simulink model "WT_FAST_09_07_2023_Afzalian"  (R2015b)
settings: Solver=FixedStepAuto  StartTime=0.0  StopTime=TMax  FixedStep=DT  MaxStep=DT  RelTol=1e-3
undefined symbols (not defined in the file): NDOF, NumOuts, q_init, qdot_init, TMax, wn, wn_A, wn_H, wn_P, zeta, zeta_A, zeta_H, zeta_P
settings Model: Creator=bjonkman  LastModifiedBy=SBU
settings SolverCC: AlgebraicLoopSolver=LineSearch
settings DataIOCC: LimitDataPoints=off  SaveFormat=Array  SignalLoggingSaveFormat=ModelDataLogs  SaveOutput=off  SaveTime=off  SignalLoggingName=sigsOut
settings OptimizationCC: ExpressionDepthLimit=2147483647
settings DebuggingCC: SaveWithParameterizedLinksMsg=none  UnderspecifiedInitializationDetection=Classic  MergeDetectMultiDrivingBlocksExec=none  SignalResolutionControl=TryResolveAllWithWarning  MultiTaskDSMMsg=warning  MultiTaskCondExecSysMsg=none  FcnCallInpInsideContextMsg=UseLocalSettings  StateNameClashWarn=warning
settings HardwareCC: ProdBitPerPointer=32  ProdLargestAtomicFloat=None  ProdIntDivRoundTo=Undefined  ProdEndianess=Unspecified  ProdWordSize=32  ProdHWDeviceType=32-bit Generic  TargetUnknown=on
settings GRTTargetCC: ModelReferenceCompliant=off  ParMdlRefBuildCompliant=off  CompOptLevelCompliant=off  ConcurrentExecutionCompliant=off  GeneratePreprocessorConditionals=Disable all  CombineOutputUpdateFcns=off  MatFileLogging=off  MATLABClassNameForMDSCustomization=Simulink.SoftwareTarget.TargetSpecificTriggerConfigurationBase  GRTInterface=on
settings ConfigComp: CovModelRefEnable=Off  CovSFcnEnable=off

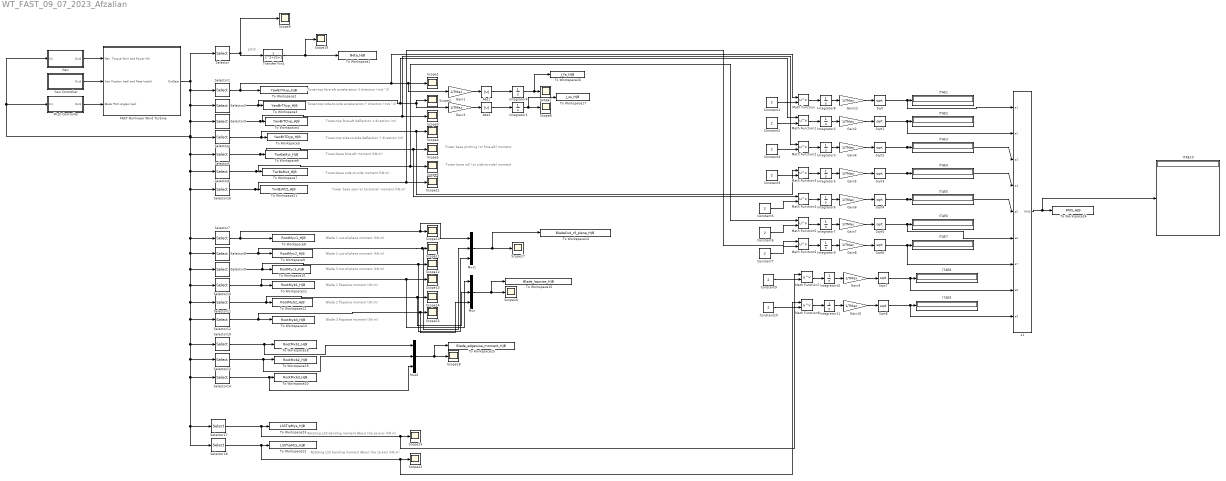
== system WT_FAST_09_07_2023_Afzalian ==
  note: Tower base yaw (or torsional) moment (kN.m)
  note: Tower base pitching (or fore-aft) moment
  note: Tower base roll (or side-to-side) moment
  note: Tower-base side-to-side moment (kN.m)
  note: Tower-base fore-aft moment (kN.m)
  note: Tower-top side-to-side deflection Y direction (m)
  note: Tower-top fore-aft deflection X direction (m)
  note: pitch
  note: Tower-top fore-aft acceleration X direction (m/s^2)
  note: Tower-top side-to-side acceleration Y direction (m/s^2)
  note: Blade 3 flapwise moment (kN.m)
  note: Blade 2 flapwise moment (kN.m)
  note: Blade 1 flapwise moment (kN.m)
  note: Blade 3 out-of-plane moment (kN.m)
  note: Blade 1 out-of-plane moment (kN.m)
  note: Blade 2 out-of-plane moment (kN.m)
  note: Rotating LSS bending moment About the ya-axis (kN.m)
  note: Rotating LSS bending moment About the za-axis (kN.m)
  Abs1 : Abs
  Abs2 : Abs
  Constant{1..7,9..10} (9 alike) : Constant  Value=2
  FAST Nonlinear Wind Turbine : Subsystem  mask(FAST Nonlinear Wind Turbine){}
      mask help: This block contains the FAST S-Function and blocks that integrate the DOF accelerations to get velocities and displacements.
      mask init:
      | clear FAST_SFunc
  Gain{1..10,12} (11 alike) : Gain  Gain=1/TMax
  Gen : Subsystem
  ITAE{1..10} (10 alike) : Display
  Integrator1 : Integrator  UpperSaturationLimit=5  LowerSaturationLimit=-5
  Integrator{2..3,5..11} (9 alike) : Integrator  UpperSaturationLimit=0.2  LowerSaturationLimit=-0.2
  Integrator4 : Integrator  UpperSaturationLimit=5  LowerSaturationLimit=-5
  Math Function{,1..8} (9 alike) : Math  Operator=pow  SaturateOnIntegerOverflow=on
  Mux : Mux  Inputs=3
  Mux1 : Mux  Inputs=3
  Mux2 : Mux  Inputs=3
  Pitch Controller : Subsystem
  Scope{1..19,21..23} (22 alike) : Scope
  Selector : Selector  InputPortWidth=48  IndexOptions=Index vector (dialog)  Indices=[9]  OutputSizes=1
  Selector1 : Selector  InputPortWidth=48  IndexOptions=Index vector (dialog)  Indices=[31]  OutputSizes=1
  Selector10 : Selector  InputPortWidth=48  IndexOptions=Index vector (dialog)  Indices=[41]  OutputSizes=1
  Selector11 : Selector  InputPortWidth=48  IndexOptions=Index vector (dialog)  Indices=[42]  OutputSizes=1
  Selector12 : Selector  InputPortWidth=48  IndexOptions=Index vector (dialog)  Indices=[43]  OutputSizes=1
  Selector13 : Selector  InputPortWidth=48  IndexOptions=Index vector (dialog)  Indices=[45]  OutputSizes=1
  Selector14 : Selector  InputPortWidth=48  IndexOptions=Index vector (dialog)  Indices=[46]  OutputSizes=1
  Selector16 : Selector  InputPortWidth=48  IndexOptions=Index vector (dialog)  Indices=[37]  OutputSizes=1
  Selector17 : Selector  InputPortWidth=48  IndexOptions=Index vector (dialog)  Indices=[44]  OutputSizes=1
  Selector18 : Selector  InputPortWidth=48  IndexOptions=Index vector (dialog)  Indices=[45]  OutputSizes=1
  Selector19 : Selector  InputPortWidth=48  IndexOptions=Index vector (dialog)  Indices=[44]  OutputSizes=1
  Selector2 : Selector  InputPortWidth=48  IndexOptions=Index vector (dialog)  Indices=[32]  OutputSizes=1
  Selector3 : Selector  InputPortWidth=48  IndexOptions=Index vector (dialog)  Indices=[33]  OutputSizes=1
  Selector4 : Selector  InputPortWidth=48  IndexOptions=Index vector (dialog)  Indices=[34]  OutputSizes=1
  Selector5 : Selector  InputPortWidth=48  IndexOptions=Index vector (dialog)  Indices=[35]  OutputSizes=1
  Selector6 : Selector  InputPortWidth=48  IndexOptions=Index vector (dialog)  Indices=[36]  OutputSizes=1
  Selector7 : Selector  InputPortWidth=48  IndexOptions=Index vector (dialog)  Indices=[38]  OutputSizes=1
  Selector8 : Selector  InputPortWidth=48  IndexOptions=Index vector (dialog)  Indices=[39]  OutputSizes=1
  Selector9 : Selector  InputPortWidth=48  IndexOptions=Index vector (dialog)  Indices=[40]  OutputSizes=1
  Sqrt{,1..8} (9 alike) : Sqrt  SaturateOnIntegerOverflow=on
  To Workspace1 : ToWorkspace  VariableName=Beta_HJB  SaveFormat=Structure With Time  SampleTime=-1
  To Workspace10 : ToWorkspace  VariableName=RootMyc3_HJB  SaveFormat=Structure With Time  SampleTime=-1
  To Workspace11 : ToWorkspace  VariableName=RootMyb1_HJB  SaveFormat=Structure With Time  SampleTime=-1
  To Workspace12 : ToWorkspace  VariableName=RootMyb2_HJB  SaveFormat=Structure With Time  SampleTime=-1
  To Workspace13 : ToWorkspace  VariableName=RootMyb3_HJB  SaveFormat=Structure With Time  SampleTime=-1
  To Workspace14 : ToWorkspace  VariableName=BladeOut_of_plane_HJB  SaveFormat=Structure With Time  SampleTime=-1
  To Workspace15 : ToWorkspace  VariableName=Blade_lapwise_HJB  SaveFormat=Structure With Time  SampleTime=-1
  To Workspace16 : ToWorkspace  VariableName=J_fa_HJB  SaveFormat=Structure With Time  SampleTime=-1
  To Workspace17 : ToWorkspace  VariableName=J_ss_HJB  SaveFormat=Structure With Time  SampleTime=-1
  To Workspace18 : ToWorkspace  VariableName=RootMxb1_HJB  SaveFormat=Structure With Time  SampleTime=-1
  To Workspace19 : ToWorkspace  VariableName=RootMxb2_HJB  SaveFormat=Structure With Time  SampleTime=-1
  To Workspace2 : ToWorkspace  VariableName=YawBrTAxp_HJB  SaveFormat=Structure With Time  SampleTime=-1
  To Workspace20 : ToWorkspace  VariableName=RootMxb3_HJB  SaveFormat=Structure With Time  SampleTime=-1
  To Workspace21 : ToWorkspace  VariableName=TwrBsMzt_HJB  SaveFormat=Structure With Time  SampleTime=-1
  To Workspace22 : ToWorkspace  VariableName=LSSTipMzs_HJB  SaveFormat=Structure With Time  SampleTime=-1
  To Workspace23 : ToWorkspace  VariableName=LSSTipMys_HJB  SaveFormat=Structure With Time  SampleTime=-1
  To Workspace24 : ToWorkspace  VariableName=RMS_HJB  SaveFormat=Structure With Time  SampleTime=-1
  To Workspace25 : ToWorkspace  VariableName=Blade_edgewise_moment_HJB  SaveFormat=Structure With Time  SampleTime=-1
  To Workspace3 : ToWorkspace  VariableName=YawBrTAyp_HJB  SaveFormat=Structure With Time  SampleTime=-1
  To Workspace4 : ToWorkspace  VariableName=YawBrTDxp_HJB  SaveFormat=Structure With Time  SampleTime=-1
  To Workspace5 : ToWorkspace  VariableName=YawBrTDyp_HJB  SaveFormat=Structure With Time  SampleTime=-1
  To Workspace6 : ToWorkspace  VariableName=TwrBsMyt_HJB  SaveFormat=Structure With Time  SampleTime=-1
  To Workspace7 : ToWorkspace  VariableName=TwrBsMxt_HJB  SaveFormat=Structure With Time  SampleTime=-1
  To Workspace8 : ToWorkspace  VariableName=RootMyc1_HJB  SaveFormat=Structure With Time  SampleTime=-1
  To Workspace9 : ToWorkspace  VariableName=RootMyc2_HJB  SaveFormat=Structure With Time  SampleTime=-1
  Transfer Fcn1 : TransferFcn
  Yaw Controller : Subsystem
  s1 : MATLAB Function  TreatAsAtomicUnit=on
  wires:
  Yaw Controller/1(Out1) -> FAST Nonlinear Wind Turbine/2(Yaw Position (rad) and Rate (rad/s))
  Pitch Controller/1(Out1) -> FAST Nonlinear Wind Turbine/3(Blade Pitch Angles (rad))
  Gen/1(Out1) -> FAST Nonlinear Wind Turbine/1(Gen. Torque (Nm) and Power (W))
  Selector9/1 -> To Workspace10/1, Mux1/3, Scope12/1
  Selector10/1 -> To Workspace11/1, Mux/1, Scope13/1
  Selector12/1 -> To Workspace13/1, Mux/3, Scope15/1
  Selector8/1 -> To Workspace9/1, Mux1/2, Scope11/1
  Selector7/1 -> To Workspace8/1, Mux1/1, Scope10/1
  Selector11/1 -> To Workspace12/1, Mux/2, Scope14/1
  Mux/1 -> To Workspace15/1, Scope16/1
  Mux1/1 -> To Workspace14/1, Scope17/1
  Abs1/1 -> Integrator4/1
  Abs2/1 -> Integrator1/1
  Integrator1/1 -> To Workspace17/1, Scope8/1
  Integrator4/1 -> To Workspace16/1, Scope7/1
  Gain1/1 -> Abs1/1
  Gain3/1 -> Abs2/1
  Selector18/1 -> To Workspace22/1, Math Function8/1, Scope22/1
  Selector17/1 -> Math Function7/1, Scope23/1, To Workspace23/1
  Selector4/1 -> Math Function3/1, Scope4/1, To Workspace5/1
  Selector5/1 -> Math Function4/1, Scope5/1, To Workspace6/1
  Selector1/1 -> Math Function/1, Gain1/1, Scope1/1, To Workspace2/1
  Math Function/1 -> Integrator8/1
  Constant1/1 -> Math Function/2
  Integrator8/1 -> Gain12/1
  Gain12/1 -> Sqrt/1
  Selector2/1 -> Math Function1/1, Gain3/1, Scope2/1, To Workspace3/1
  Math Function1/1 -> Integrator2/1
  Constant2/1 -> Math Function1/2
  Integrator2/1 -> Gain2/1
  Gain2/1 -> Sqrt1/1
  Selector3/1 -> Math Function2/1, Scope3/1, To Workspace4/1
  Math Function2/1 -> Integrator3/1
  Constant4/1 -> Math Function2/2
  Integrator3/1 -> Gain4/1
  Gain4/1 -> Sqrt2/1
  Math Function3/1 -> Integrator5/1
  Constant3/1 -> Math Function3/2
  Integrator5/1 -> Gain5/1
  Gain5/1 -> Sqrt3/1
  Constant5/1 -> Math Function4/2
  Gain6/1 -> Sqrt4/1
  Selector6/1 -> Math Function5/1, Scope6/1, To Workspace7/1
  Constant6/1 -> Math Function5/2
  Gain7/1 -> Sqrt5/1
  Integrator7/1 -> Gain7/1
  Integrator6/1 -> Gain6/1
  Math Function4/1 -> Integrator6/1
  Math Function5/1 -> Integrator7/1
  Selector16/1 -> Math Function6/1, Scope21/1, To Workspace21/1
  Constant7/1 -> Math Function6/2
  Gain8/1 -> Sqrt6/1
  Integrator9/1 -> Gain8/1
  Math Function6/1 -> Integrator9/1
  Sqrt/1 -> s1/1(a1), ITAE1/1
  Sqrt1/1 -> s1/2(a2), ITAE2/1
  Sqrt2/1 -> s1/3(a3), ITAE3/1
  Sqrt3/1 -> s1/4(a4), ITAE4/1
  Sqrt4/1 -> s1/5(a5), ITAE5/1
  Sqrt6/1 -> s1/7(a7), ITAE7/1
  s1/1(RMS) -> ITAE10/1, To Workspace24/1
  Sqrt5/1 -> s1/6(a6), ITAE6/1
  Constant9/1 -> Math Function7/2
  Gain9/1 -> Sqrt7/1
  Integrator10/1 -> Gain9/1
  Math Function7/1 -> Integrator10/1
  Sqrt7/1 -> s1/8(a8), ITAE8/1
  Constant10/1 -> Math Function8/2
  Gain10/1 -> Sqrt8/1
  Integrator11/1 -> Gain10/1
  Math Function8/1 -> Integrator11/1
  Sqrt8/1 -> s1/9(a9), ITAE9/1
  FAST Nonlinear Wind Turbine/1(OutData) -> Selector16/1, Selector19/1, Selector13/1, Selector14/1, Selector18/1, Selector17/1, Selector12/1, Selector11/1, Selector10/1, Selector9/1, Selector8/1, Selector7/1, Selector6/1, Selector5/1, Selector4/1, Gen/1(In1), Pitch Controller/1(In1), Selector3/1, Selector2/1, Selector1/1, Selector/1
  Selector19/1 -> Mux2/1, To Workspace18/1
  Selector13/1 -> Mux2/2, To Workspace19/1
  Selector14/1 -> Mux2/3, To Workspace20/1
  Mux2/1 -> Scope18/1, To Workspace25/1
  Selector/1 -> Transfer Fcn1/1, Scope9/1
  Transfer Fcn1/1 -> Scope19/1, To Workspace1/1

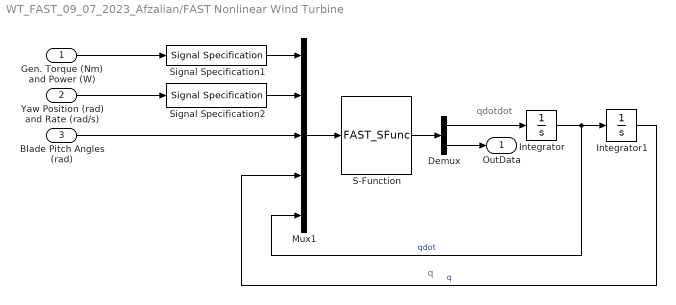
== system WT_FAST_09_07_2023_Afzalian/FAST Nonlinear Wind Turbine ==
  note: qdotdot
  note: q
  Gen. Torque (Nm) and Power (W) : Inport
  Yaw Position (rad) and Rate (rad/s) : Inport  Port=2
  Blade Pitch Angles (rad) : Inport  Port=3
  Demux : Demux  Outputs=[NDOF, NumOuts]
  Integrator : Integrator  InitialCondition=qdot_init
  Integrator1 : Integrator  InitialCondition=q_init
  Mux1 : Mux  Inputs=5
  S-Function : S-Function  FunctionName=FAST_SFunc  SFunctionDeploymentMode=off  EnableBusSupport=off
  Signal Specification1 : SignalSpecification  OutDataTypeStr=double  Dimensions=2
  Signal Specification2 : SignalSpecification  OutDataTypeStr=double  Dimensions=2
  OutData : Outport
  wires:
  Integrator/1 -> Integrator1/1, Mux1/5  "qdot"
  Gen. Torque (Nm) and Power (W)/1 -> Signal Specification1/1
  S-Function/1 -> Demux/1
  Demux/1 -> Integrator/1
  Demux/2 -> OutData/1
  Mux1/1 -> S-Function/1
  Blade Pitch Angles (rad)/1 -> Mux1/3
  Yaw Position (rad) and Rate (rad/s)/1 -> Signal Specification2/1
  Integrator1/1 -> Mux1/4  "q"
  Signal Specification1/1 -> Mux1/1
  Signal Specification2/1 -> Mux1/2

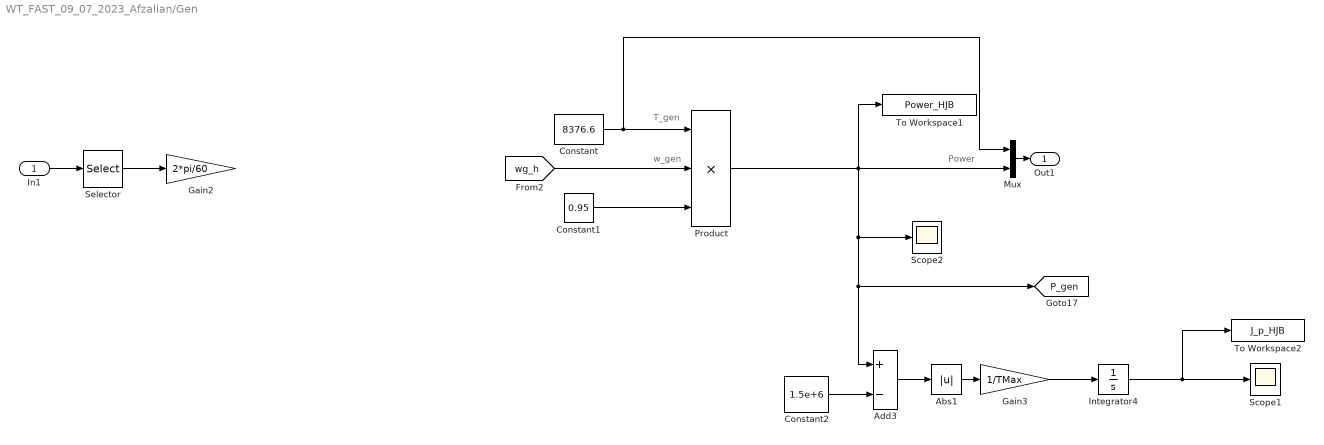
== system WT_FAST_09_07_2023_Afzalian/Gen ==
  note: T_gen
  note: w_gen
  note: Power
  In1 : Inport
  Abs1 : Abs
  Add3 : Sum  Inputs=+-
  Constant : Constant  Value=8376.6
  Constant1 : Constant  Value=0.95
  Constant2 : Constant  Value=1.5e+6
  Gain2 : Gain  Gain=2*pi/60
  Gain3 : Gain  Gain=1/TMax
  Integrator4 : Integrator  UpperSaturationLimit=5  LowerSaturationLimit=-5
  Mux : Mux  Inputs=2
  Product : Product  Inputs=3
  Scope1 : Scope
  Scope2 : Scope
  Selector : Selector  InputPortWidth=48  IndexOptions=Index vector (dialog)  Indices=[25]  OutputSizes=1
  To Workspace1 : ToWorkspace  VariableName=Power_HJB  SaveFormat=Structure With Time  SampleTime=-1
  To Workspace2 : ToWorkspace  VariableName=J_p_HJB  SaveFormat=Structure With Time  SampleTime=-1
  Out1 : Outport
  tag scope: P_gen=global
  wires:
  Constant1/1 -> Product/3
  Constant/1 -> Mux/1, Product/1
  In1/1 -> Selector/1
  Selector/1 -> Gain2/1
  Product/1 -> To Workspace1/1, Mux/2, Add3/1, [P_gen], Scope2/1
  Constant2/1 -> Add3/2
  Add3/1 -> Abs1/1
  Integrator4/1 -> Scope1/1, To Workspace2/1
  Gain3/1 -> Integrator4/1
  Abs1/1 -> Gain3/1
  Mux/1 -> Out1/1
  [wg_h] -> Product/2

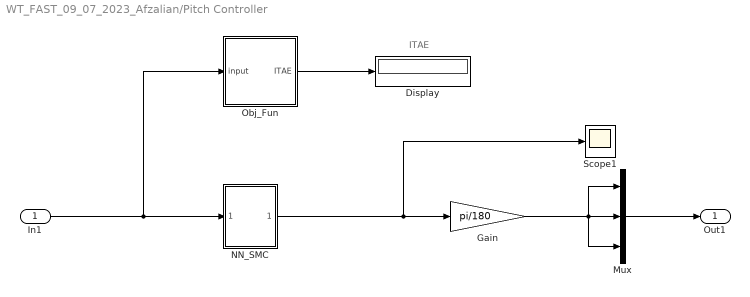
== system WT_FAST_09_07_2023_Afzalian/Pitch Controller ==
  note: ITAE
  In1 : Inport
  Display : Display
  Gain : Gain  Gain=pi/180
  Mux : Mux  Inputs=3
  NN_SMC : Subsystem
  Obj_Fun : Subsystem
  Scope1 : Scope
  Out1 : Outport
  wires:
  In1/1 -> NN_SMC/1(input), Obj_Fun/1("input ")
  Obj_Fun/1(ITAE) -> Display/1
  Mux/1 -> Out1/1
  Gain/1 -> Mux/3, Mux/1, Mux/2
  NN_SMC/1(Out1) -> Scope1/1, Gain/1

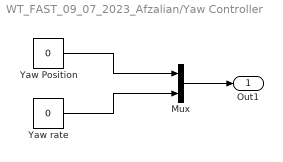
== system WT_FAST_09_07_2023_Afzalian/Yaw Controller ==
  Mux : Mux  Inputs=2
  Yaw Position : Constant  Value=0
  Yaw rate : Constant  Value=0
  Out1 : Outport
  wires:
  Mux/1 -> Out1/1
  Yaw Position/1 -> Mux/1
  Yaw rate/1 -> Mux/2

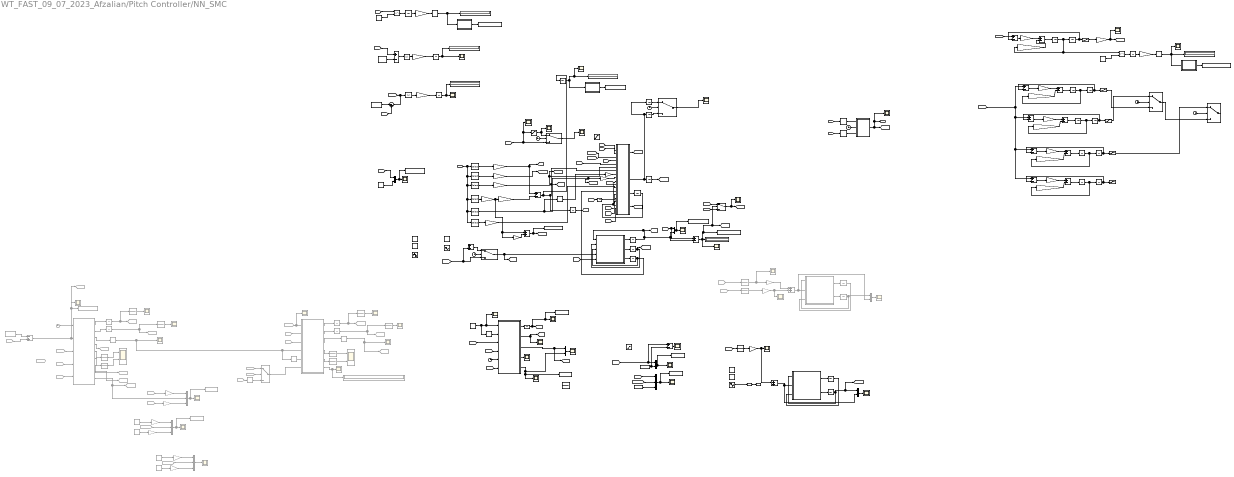
== system WT_FAST_09_07_2023_Afzalian/Pitch Controller/NN_SMC ==
  note: Step 1
  note: wind
  note: deltadot
  note: wgen
  note: xdot2
  note: xdot1
  note: w_rotor
  note: Step 2
  note: Stress
  note: J_P
  note: RMSE
  note: J_w
  input : Inport
  Abs1 : Abs
  Abs6 : Abs
  Add{,1,4,7,9..13,15..19} (14 alike) : Sum  Inputs=+-
  Add14 : Sum
  Add2 : Sum  Commented=on
  Add3 : Sum
  Add5 : Sum
  Add6 : Sum  Commented=on  Inputs=-+
  Clock{1..2,4..8} (7 alike) : Clock
  Clock3 : Clock  Commented=on
  Constant10 : Constant
  Constant11 : Constant  Value=rand
  Constant12 : Constant  Value=0.5
  Constant13 : Constant
  Constant14 : Constant  Value=1.5e6
  Constant15 : Constant
  Constant2 : Constant  Value=2
  Constant3 : Constant  Value=2
  Constant4 : Constant  Value=rand
  Constant5 : Constant  Commented=on  Value=1.5
  Constant6 : Constant  Commented=on  Value=0.5
  Constant7 : Constant  Commented=on  Value=0.5
  Constant8 : Constant  Commented=on  Value=1.5
  Constant9 : Constant  Value=1.5e+6
  D_hat : MATLAB Function  Commented=on  TreatAsAtomicUnit=on
  D_hat1 : MATLAB Function  TreatAsAtomicUnit=on
  Delay : Delay  DelayLength=1  InitialCondition=0
  Delay1 : Delay  DelayLength=1  InitialCondition=0
  Derivative{,1..2,4} (4 alike) : Derivative
  Derivative3 : Derivative  Commented=on
  Display : Display
  From14 : From  Commented=on  GotoTag=W_c  TagVisibility=global
  From15 : From  Commented=on  GotoTag=WWW  TagVisibility=global
  From17 : From  Commented=on  GotoTag=V  TagVisibility=global
  From31 : From  Commented=on  GotoTag=xdot1  TagVisibility=global
  From32 : From  Commented=on  GotoTag=W_a  TagVisibility=global
  From33 : From  Commented=on  GotoTag=W2_c  TagVisibility=global
  From35 : From  Commented=on  GotoTag=Res  TagVisibility=global
  From36 : From  Commented=on  GotoTag=wdotr_hat  TagVisibility=global
  From37 : From  Commented=on  GotoTag=wdotr_hat  TagVisibility=global
  From38 : From  Commented=on  GotoTag=rho_U  TagVisibility=global
  From39 : From  Commented=on  GotoTag=EE  TagVisibility=global
  From40 : From  Commented=on  GotoTag=W2_a  TagVisibility=global
  From41 : From  Commented=on  GotoTag=F_h  TagVisibility=global
  From42 : From  Commented=on  GotoTag=Lf  TagVisibility=global
  From44 : From  Commented=on  GotoTag=rho_L  TagVisibility=global
  From45 : From  Commented=on  GotoTag=EE  TagVisibility=global
  From6 : From  Commented=on  GotoTag=Lf  TagVisibility=global
  Gain : Gain  Gain=2*pi/60
  Gain1 : Gain  Gain=pi/180
  Gain{5,8,10,25} (4 alike) : Gain  Commented=on
  Gain{11,17,19..20} (4 alike) : Gain
  Gain{12,14..15,23} (4 alike) : Gain  Gain=1/TMax
  Gain13 : Gain  Gain=2*zeta*wn
  Gain16 : Gain  Gain=0.01
  Gain18 : Gain  Commented=on  Gain=0.3
  Gain2 : Gain  Gain=pi/180
  Gain21 : Gain  Commented=on  Gain=-1
  Gain22 : Gain  Commented=on  Gain=-1
  Gain24 : Gain  Commented=on  Gain=-1
  Gain26 : Gain  Gain=2*zeta_A*wn_A
  Gain27 : Gain  Gain=wn_P
  Gain28 : Gain  Gain=2*zeta_P*wn_P
  Gain29 : Gain  Gain=wn
  Gain3 : Gain  Gain=2*pi/60
  Gain30 : Gain  Gain=2*zeta*wn
  Gain31 : Gain  Gain=wn_H
  Gain32 : Gain  Gain=2*zeta_H*wn_H
  Gain4 : Gain  Gain=1/87.965
  Gain6 : Gain  Gain=1000
  Gain7 : Gain  Gain=wn
  Gain9 : Gain  Gain=wn_A
  Goto15 : Goto  Commented=on  GotoTag=W2_a  TagVisibility=global
  Goto16 : Goto  Commented=on  GotoTag=W_a  TagVisibility=global
  Goto2 : Goto  Commented=on  GotoTag=S  TagVisibility=global
  Goto23 : Goto  Commented=on  GotoTag=EE  TagVisibility=global
  Goto24 : Goto  Commented=on  GotoTag=YY  TagVisibility=global
  Goto25 : Goto  Commented=on  GotoTag=rho_U  TagVisibility=global
  Goto26 : Goto  Commented=on  GotoTag=W2_c  TagVisibility=global
  Goto27 : Goto  Commented=on  GotoTag=rho_L  TagVisibility=global
  Goto28 : Goto  Commented=on  GotoTag=W_c  TagVisibility=global
  Goto29 : Goto  Commented=on  GotoTag=e_1  TagVisibility=global
  ITAE{1,3..6} (5 alike) : Display
  ITAE2 : Display  Commented=on
  Integrator1 : Integrator  UpperSaturationLimit=5  LowerSaturationLimit=-5
  Integrator{8..10,14} (4 alike) : Integrator  Commented=on  InitialCondition=0.1  UpperSaturationLimit=10  LowerSaturationLimit=-10
  Integrator11 : Integrator  Commented=on  InitialCondition=0.1
  Integrator12 : Integrator  InitialCondition=0.1  LimitOutput=on  UpperSaturationLimit=100  LowerSaturationLimit=-100
  Integrator13 : Integrator  InitialCondition=0.1  UpperSaturationLimit=10  LowerSaturationLimit=-10
  Integrator{2,6,15,25,27,29} (6 alike) : Integrator  UpperSaturationLimit=90  LowerSaturationLimit=-1
  Integrator16 : Integrator  InitialCondition=2.1428
  Integrator17 : Integrator  Commented=on  InitialCondition=0.1
  Integrator18 : Integrator
  Integrator{19,26,28,30..31} (5 alike) : Integrator  LimitOutput=on  UpperSaturationLimit=8  LowerSaturationLimit=-8
  Integrator20 : Integrator  UpperSaturationLimit=0.2  LowerSaturationLimit=-0.2
  Integrator21 : Integrator  UpperSaturationLimit=0.2  LowerSaturationLimit=-0.2
  Integrator22 : Integrator  InitialCondition=180  LimitOutput=on  UpperSaturationLimit=200  LowerSaturationLimit=170
  Integrator23 : Integrator
  Integrator24 : Integrator  UpperSaturationLimit=5  LowerSaturationLimit=-5
  Integrator3 : Integrator  InitialCondition=2.1428  UpperSaturationLimit=2.5
  Integrator32 : Integrator  InitialCondition=0.1  UpperSaturationLimit=500  LowerSaturationLimit=-500
  Integrator33 : Integrator  UpperSaturationLimit=200
  Integrator4 : Integrator  UpperSaturationLimit=0.2  LowerSaturationLimit=-0.2
  Integrator5 : Integrator  UpperSaturationLimit=10  LowerSaturationLimit=-10
  Integrator7 : Integrator  InitialCondition=0.3
  Math Function1 : Math  Operator=pow  SaturateOnIntegerOverflow=on
  Math Function2 : Math  Operator=pow  SaturateOnIntegerOverflow=on
  Memory2 : Memory  Commented=on
  Memory3 : Memory  Commented=on
  Memory4 : Memory  Commented=on
  Mux{,1,4..5,9} (5 alike) : Mux  Inputs=2
  Mux2 : Mux  Commented=on  Inputs=2
  Mux3 : Mux  Inputs=3
  Mux6 : Mux  Commented=on  Inputs=3
  Mux7 : Mux  Commented=on  Inputs=3
  Mux8 : Mux  Commented=on  Inputs=3
  Observer1 : MATLAB Function  TreatAsAtomicUnit=on
  Observer2 : MATLAB Function  TreatAsAtomicUnit=on
  Observer3 : MATLAB Function  TreatAsAtomicUnit=on
  Observer4 : MATLAB Function  TreatAsAtomicUnit=on
  SMC : MATLAB Function  TreatAsAtomicUnit=on
  Saturation{1,4..7} (5 alike) : Saturate  UpperLimit=90  LowerLimit=-1
  Saturation2 : Saturate  UpperLimit=2.2  LowerLimit=-2.2
  Saturation3 : Saturate  UpperLimit=2.2  LowerLimit=-2.2
  Saturation9 : Saturate  UpperLimit=200  LowerLimit=-200
  Scope{1..4,6..7,9} (7 alike) : Scope
  Selector : Selector  InputPortWidth=48  IndexOptions=Index vector (dialog)  Indices=[24]  OutputSizes=1
  Selector1 : Selector  InputPortWidth=48  IndexOptions=Index vector (dialog)  Indices=[29]  OutputSizes=1
  Selector2 : Selector  InputPortWidth=48  IndexOptions=Index vector (dialog)  Indices=[30]  OutputSizes=1
  Selector3 : Selector  InputPortWidth=48  IndexOptions=Index vector (dialog)  Indices=[25]  OutputSizes=1
  Selector4 : Selector  InputPortWidth=48  IndexOptions=Index vector (dialog)  Indices=[26]  OutputSizes=1
  Selector5 : Selector  InputPortWidth=48  IndexOptions=Index vector (dialog)  Indices=[28]  OutputSizes=1
  Sine Wave1 : Sin  Amplitude=0.25  Bias=0.25  Frequency=pi/40  SampleTime=0
  Sine Wave2 : Sin  Amplitude=0.5  Bias=0.2  Frequency=pi/20  SampleTime=0
  Sine Wave5 : Sin  Amplitude=0.5  Bias=0.25  Frequency=pi/40  SampleTime=0
  Sqrt1 : Sqrt  SaturateOnIntegerOverflow=on
  Sqrt2 : Sqrt  SaturateOnIntegerOverflow=on
  Sum : Sum  Inputs=|-+
  Switch : Switch  Threshold=0.05
  Switch1 : Switch  Threshold=80
  Switch2 : Switch  Threshold=100
  Switch3 : Switch  Threshold=100
  Switch4 : Switch  Threshold=100
  Switch5 : Switch  Commented=on  Threshold=0.0005
  Switch6 : Switch  Threshold=180
  To Workspace1 : ToWorkspace  Commented=on  VariableName=E_BLF  SaveFormat=Structure With Time  SampleTime=-1
  To Workspace10 : ToWorkspace  VariableName=Q_RL  SaveFormat=Structure With Time  SampleTime=-1
  To Workspace11 : ToWorkspace  VariableName=P_gen_HJB  SaveFormat=Structure With Time  SampleTime=-1
  To Workspace12 : ToWorkspace  VariableName=wg_HJB  SaveFormat=Structure With Time  SampleTime=-1
  To Workspace13 : ToWorkspace  VariableName=RMS_Beta_HJB  SaveFormat=Structure With Time  SampleTime=-1
  To Workspace14 : ToWorkspace  VariableName=Ka_RL  SaveFormat=Structure With Time  SampleTime=-1
  To Workspace2 : ToWorkspace  VariableName=wr_est_HJB  SaveFormat=Structure With Time  SampleTime=-1
  To Workspace3 : ToWorkspace  VariableName=RES  SaveFormat=Structure With Time  SampleTime=-1
  To Workspace4 : ToWorkspace  VariableName=S_HJB  SaveFormat=Structure With Time  SampleTime=-1
  To Workspace5 : ToWorkspace  Commented=on  VariableName=PP  SaveFormat=Structure With Time  SampleTime=-1
  To Workspace6 : ToWorkspace  VariableName=wr_HJB  SaveFormat=Structure With Time  SampleTime=-1
  To Workspace7 : ToWorkspace  VariableName=RMS_wr_HJB  SaveFormat=Structure With Time  SampleTime=-1
  To Workspace8 : ToWorkspace  VariableName=Pg_HJB  SaveFormat=Structure With Time  SampleTime=-1
  To Workspace9 : ToWorkspace  Commented=on  VariableName=PP1  SaveFormat=Structure With Time  SampleTime=-1
  Transfer Fcn{1..6,8..11} (10 alike) : TransferFcn  Commented=on
  Transfer Fcn13 : TransferFcn
  Transfer Fcn7 : TransferFcn
  W_rotor_rarted1 : Constant  Value=2.1428
  W_rotor_rarted2 : Constant  Value=2.1428
  W_rotor_rarted3 : Constant  Value=1.5e6
  W_rotor_rarted4 : Constant  Commented=on  Value=2.1428
  s1 : MATLAB Function  TreatAsAtomicUnit=on
  s2 : MATLAB Function  Commented=on  TreatAsAtomicUnit=on
  s3 : MATLAB Function  TreatAsAtomicUnit=on
  s4 : MATLAB Function  Commented=on  TreatAsAtomicUnit=on
  wr_est{1..4,9,14..17,21,24..25,29,31..35} (18 alike) : Scope
  wr_est{5..7,10..13,18..20,22,26..28,30} (15 alike) : Scope  Commented=on
  wr_est23 : Scope  Commented=on  NumInputPorts=2
  wr_est8 : Scope  Commented=on  NumInputPorts=2
  Out1 : Outport
  tag scope: F_h=global, K=global, Ka=global, Lf=global, Res=global, V=global, WWW=global, W_At=global, delta=global, deltadot=global, e=global, rd_hat=global, u1=global, uu=global, uuu=global, wdotg=global, wdotr_hat=global, wg=global, wg_h=global, wr=global, wr_hat=global, xdot1=global
  wires:
  W_rotor_rarted1/1 -> Sum/1
  Selector/1 -> Gain/1
  Selector1/1 -> Gain1/1
  Selector2/1 -> Gain2/1
  input/1 -> Selector5/1, Selector4/1, Selector3/1, Selector2/1, Selector1/1, Selector/1
  Selector3/1 -> Gain3/1
  Gain4/1 -> Add/2
  Selector5/1 -> Gain6/1
  Gain1/1 -> [xdot1]
  Gain2/1 -> [wdotg], SMC/6(wdotg)
  Add/1 -> Integrator2/1, Integrator7/1, [deltadot], SMC/7(deltadot)
  Gain6/1 -> SMC/12(Pr)
  Derivative/1 -> Gain17/1
  Selector4/1 -> Derivative/1, [V], Gain11/1
  [uuu] -> SMC/5(Beta)
  [wg_h] -> SMC/10(wg)
  s1/2(zhatdot2) -> Integrator4/1
  s1/3(zhatdot3) -> Integrator5/1
  Integrator4/1 -> [wdotr_hat], s1/2(zhat2)
  Integrator5/1 -> s1/3(zhat3), SMC/13(psihat)
  Mux/1 -> Scope1/1, To Workspace2/1
  Add1/1 -> Switch/2, [Res], To Workspace3/1, wr_est1/1, Display/1
  [uuu] -> s1/5(u)
  [wr] -> Add1/1, Mux/1
  Integrator7/1 -> [delta]
  Abs6/1 -> Gain12/1
  Integrator1/1 -> Scope7/1, ITAE3/1
  Gain12/1 -> Integrator1/1
  Sum/1 -> [e], Abs6/1
  [e] -> Integrator16/1
  Integrator16/1 -> SMC/14(inte)
  [e] -> SMC/2(e)
  [wdotr_hat] -> SMC/3(xdot1)
  SMC/3(Wg_dot) -> Integrator33/1, Integrator22/1, Integrator23/1
  SMC/4(D_dot) -> Integrator18/1
  Math Function2/1 -> Integrator21/1
  Constant3/1 -> Math Function2/2
  Integrator21/1 -> Gain15/1
  Gain15/1 -> Sqrt2/1
  Sqrt2/1 -> Scope4/1, ITAE5/1, Observer4/1(a1)
  Observer4/1(RMS_wr) -> To Workspace13/1
  Integrator2/1 -> Scope6/1, ITAE1/1, Observer1/1(a1)
  Observer1/1(RMS_wr) -> To Workspace4/1
  Add11/1 -> Gain7/1
  Gain7/1 -> Add12/1
  Gain13/1 -> Add12/2
  Add12/1 -> Integrator19/1
  Integrator19/1 -> Integrator6/1, Gain13/1, Math Function2/1
  Saturation1/1 -> Gain20/1
  Integrator6/1 -> Add11/2, Saturation1/1
  Gain20/1 -> [uu], Scope2/1
  Constant14/1 -> Mux1/2
  [P_gen] -> Mux1/1
  Mux1/1 -> To Workspace11/1, Scope3/1
  Gain3/1 -> Gain16/1, Add14/1, Gain4/1
  Add14/1 -> To Workspace12/1, [wg]
  Gain16/1 -> Add14/2
  Clock2/1 -> Switch4/2
  [wr] -> Add3/2, Switch4/3
  Add3/1 -> Switch4/1
  Switch4/1 -> [W_At], s1/4(z1)
  Integrator18/1 -> SMC/11(delta), SMC/15(DD)
  [wg_h] -> SMC/16(Wg)
  Gain11/1 -> SMC/9(V)
  Gain17/1 -> SMC/8(Vdot)
  s4/1(W_ad) -> Integrator10/1
  s4/2(W_cd) -> Integrator11/1
  From32/1 -> s4/4(W_a)
  From14/1 -> s4/5(W_c)
  s4/3(alpha_hat) -> Memory3/1
  Memory3/1 -> Derivative3/1, s2/4(alpha_hat), wr_est7/1
  Integrator11/1 -> Transfer Fcn4/1, Goto28/1
  [K] -> SMC/17(K)
  [S] -> SMC/1(S)
  s4/4(S) -> Goto2/1
  W_rotor_rarted2/1 -> Mux3/3
  W_rotor_rarted3/1 -> Add15/2, Mux4/2
  Mux3/1 -> wr_est4/1, To Workspace6/1
  Mux4/1 -> wr_est9/1, To Workspace8/1
  [wr_hat] -> Mux3/2
  [wr] -> Mux3/1
  Add15/1 -> wr_est21/1
  Integrator10/1 -> Transfer Fcn1/1, Goto16/1
  s4/5(WW_a) -> Transfer Fcn5/1
  s4/6(WW_c) -> Transfer Fcn6/1
  SMC/5(Lf) -> [Lf]
  Gain/1 -> [wr], Add/1
  D_hat/2(dhat_dot) -> Integrator8/1
  Integrator8/1 -> Mux2/1, D_hat/1(dhat)
  D_hat/1(bhat3_dot) -> Integrator9/1
  Integrator9/1 -> D_hat/3(bhat3)
  Mux2/1 -> wr_est11/1
  Add2/1 -> Mux2/2, D_hat/2(d)
  From6/1 -> Transfer Fcn3/1
  Gain10/1 -> wr_est13/1, Add2/2
  From17/1 -> Transfer Fcn2/1
  Gain18/1 -> Add2/1
  Transfer Fcn2/1 -> wr_est12/1, Gain18/1
  Transfer Fcn3/1 -> Gain10/1
  Clock4/1 -> Switch3/2
  Saturation2/1 -> Switch3/1, wr_est14/1
  Switch3/1 -> wr_est3/1
  [wr_hat] -> Switch3/3, wr_est15/1, Saturation2/1
  Transfer Fcn1/1 -> wr_est6/1
  Transfer Fcn4/1 -> wr_est5/1
  Transfer Fcn5/1 -> wr_est8/1
  Transfer Fcn6/1 -> wr_est8/2
  [uu] -> Delay1/1
  Clock1/1 -> Observer2/2(t)
  [wr] -> Delay/1
  Delay/1 -> Observer2/3(Wr)
  Observer2/1(H) -> wr_est2/1, Out1/1, [uuu]
  Delay1/1 -> Observer2/1(u)
  D_hat1/2(dhat_dot) -> Integrator12/1
  Integrator12/1 -> D_hat1/1(dhat), Mux5/1, [F_h]
  D_hat1/1(bhat3_dot) -> Integrator13/1
  Integrator13/1 -> D_hat1/3(bhat3)
  Mux5/1 -> wr_est16/1
  Derivative1/1 -> Derivative2/1
  Add5/1 -> Mux5/2, D_hat1/2(d)
  [Lf] -> Transfer Fcn7/1
  Gain19/1 -> Add5/1, wr_est17/1
  Transfer Fcn7/1 -> Gain19/1
  Switch/1 -> wr_est25/1, [WWW]
  [wr] -> Switch/1
  [wr_hat] -> Switch/3
  [u1] -> Add11/1
  SMC/1(u_RL) -> [u1]
  From36/1 -> wr_est27/1, s2/1(ed1)
  s2/1(W_ad) -> Integrator14/1
  s2/2(W_cd) -> Integrator17/1
  From40/1 -> s2/2(W_a)
  From33/1 -> s2/3(W_c)
  s2/3(U_hat) -> Memory4/1
  Memory4/1 -> wr_est22/1, Goto24/1
  Integrator17/1 -> Goto26/1, Transfer Fcn9/1
  Integrator14/1 -> Goto15/1, Transfer Fcn8/1
  s2/4(WW_a) -> Transfer Fcn10/1
  s2/5(WW_c) -> Transfer Fcn11/1
  From41/1 -> Memory2/1
  Transfer Fcn8/1 -> wr_est20/1
  Transfer Fcn9/1 -> wr_est19/1
  Transfer Fcn10/1 -> wr_est23/1
  Transfer Fcn11/1 -> wr_est23/2
  Derivative3/1 -> s2/5(alpha_dot)
  s2/6(J2) -> ITAE2/1, wr_est18/1
  [wr_hat] -> Sum/2
  From35/1 -> Switch5/2
  From42/1 -> Switch5/1
  Memory2/1 -> Switch5/3
  Switch5/1 -> s2/6(F_h)
  s1/1(zhatdot1) -> Integrator3/1
  Integrator3/1 -> Add1/2, Mux/2, [wr_hat], s1/1(zhat1)
  Add6/1 -> s4/2(e1), Goto23/1, wr_est26/1, To Workspace1/1
  From15/1 -> Add6/2
  W_rotor_rarted4/1 -> Add6/1
  From37/1 -> s4/3(ed)
  Constant8/1 -> Gain21/1
  Mux6/1 -> To Workspace5/1, wr_est28/1
  Constant5/1 -> Gain5/1
  Gain5/1 -> Mux6/1
  Gain21/1 -> Mux6/3
  From39/1 -> Mux6/2
  s4/7(rho_U) -> Goto25/1
  s4/8(rho_L) -> Goto27/1
  Clock3/1 -> s4/1(t)
  From44/1 -> Gain22/1
  Mux7/1 -> To Workspace9/1, wr_est10/1
  From38/1 -> Gain8/1
  Gain8/1 -> Mux7/1
  Gain22/1 -> Mux7/3
  s4/9(e) -> Goto29/1, Mux7/2
  Clock6/1 -> Switch2/2
  Integrator22/1 -> Switch2/1
  Integrator23/1 -> Switch2/3
  Constant9/1 -> Add7/2
  Add7/1 -> Abs1/1
  Integrator24/1 -> Scope9/1, ITAE6/1
  Gain23/1 -> Integrator24/1
  Abs1/1 -> Gain23/1
  [P_gen] -> Add7/1
  [e] -> Math Function1/1
  Math Function1/1 -> Integrator20/1
  Constant2/1 -> Math Function1/2
  Integrator20/1 -> Gain14/1
  Gain14/1 -> Sqrt1/1
  Sqrt1/1 -> Observer3/1(a1), ITAE4/1
  Observer3/1(RMS_wr) -> To Workspace7/1
  Constant7/1 -> Gain24/1
  Mux8/1 -> wr_est30/1
  Constant6/1 -> Gain25/1
  Gain25/1 -> Mux8/1
  Gain24/1 -> Mux8/3
  From45/1 -> Mux8/2
  Sine Wave5/1 -> Derivative1/1
  Add18/1 -> Gain31/1
  Gain31/1 -> Add19/1
  Gain32/1 -> Add19/2
  Add19/1 -> Integrator31/1
  Integrator31/1 -> Integrator15/1, Gain32/1
  Integrator15/1 -> Saturation4/1, Add18/2
  Saturation4/1 -> Switch1/1
  Clock7/1 -> Switch1/2
  Switch1/1 -> Switch6/3
  Add17/1 -> Gain29/1
  Gain29/1 -> Add10/1
  Gain30/1 -> Add10/2
  Add10/1 -> Integrator26/1
  Integrator26/1 -> Gain30/1, Integrator25/1
  Integrator25/1 -> Add17/2, Saturation7/1
  Saturation7/1 -> Switch1/3
  Clock5/1 -> Switch6/2
  Add9/1 -> Gain9/1
  Gain9/1 -> Add13/1
  Gain26/1 -> Add13/2
  Add13/1 -> Integrator28/1
  Integrator28/1 -> Gain26/1, Integrator27/1
  Integrator27/1 -> Add9/2, Saturation5/1
  Saturation5/1 -> Switch6/1
  Add16/1 -> Gain27/1
  Gain27/1 -> Add4/1
  Gain28/1 -> Add4/2
  Add4/1 -> Integrator30/1
  Integrator30/1 -> Integrator29/1, Gain28/1
  Integrator29/1 -> Saturation6/1, Add16/2
  [u1] -> Add16/1, Add9/1, Add18/1, Add17/1
  Clock8/1 -> s3/5(t)
  s3/1(Ka_dot) -> Integrator32/1
  Integrator32/1 -> To Workspace14/1, wr_est32/1, [Ka]
  [Ka] -> s3/6(Ka)
  s3/2(K) -> [K], wr_est33/1
  s3/5(Q) -> Mux9/2, To Workspace10/1, wr_est34/1
  s3/4(W) -> wr_est35/1
  Constant13/1 -> Derivative4/1, wr_est31/1, s3/1(eta)
  Derivative4/1 -> s3/2(eta_dot)
  Mux9/1 -> wr_est24/1
  [e] -> s3/4(e)
  s3/3(Qh) -> [rd_hat], Mux9/1
  [xdot1] -> s3/3(xdot1)
  [rd_hat] -> SMC/18(rd_hat)
  [wr_hat] -> SMC/4(wr)
  Switch2/1 -> wr_est29/1
  [P_gen] -> Add15/1, Mux4/1
  Integrator33/1 -> [wg_h]

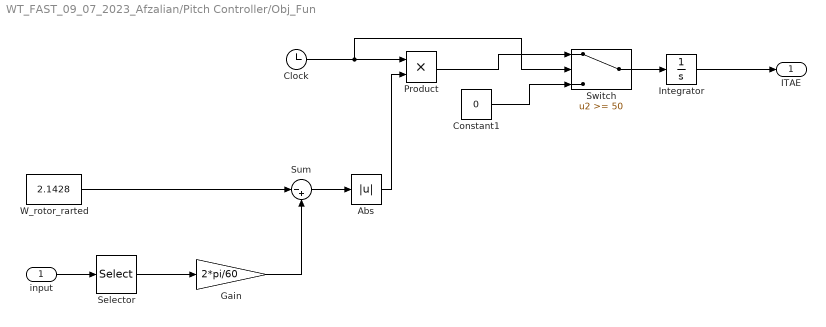
== system WT_FAST_09_07_2023_Afzalian/Pitch Controller/Obj_Fun ==
  "input " : Inport
  Abs : Abs
  Clock : Clock
  Constant1 : Constant  Value=0
  Gain : Gain  Gain=2*pi/60
  Integrator : Integrator
  Product : Product
  Selector : Selector  InputPortWidth=48  IndexOptions=Index vector (dialog)  Indices=[24]  OutputSizes=1
  Sum : Sum  Inputs=|-+
  Switch : Switch  Threshold=50
  W_rotor_rarted : Constant  Value=2.1428
  ITAE : Outport
  wires:
  Clock/1 -> Switch/2, Product/1
  Abs/1 -> Product/2
  Switch/1 -> Integrator/1
  Integrator/1 -> ITAE/1
  Constant1/1 -> Switch/3
  Product/1 -> Switch/1
  W_rotor_rarted/1 -> Sum/1
  Gain/1 -> Sum/2
  Selector/1 -> Gain/1
  "input "/1 -> Selector/1
  Sum/1 -> Abs/1

== matlab function WT_FAST_09_07_2023_Afzalian/Pitch Controller/NN_SMC/Observer3 ==
  data: a1 input; RMS_wr output
function RMS_wr  = fcn(a1)

RMS_wr = a1;

== matlab function WT_FAST_09_07_2023_Afzalian/Pitch Controller/NN_SMC/SMC ==
  data: S input; u_RL output; u_NPI output; e input; xdot1 input; Wg_dot output; D_dot output; wr input; Beta input; wdotg input; deltadot input; Vdot input; V input; wg input; delta input; Pr input; psihat input; inte input; DD input; Wg input; K input; Lf output; rd_hat input
function [u_RL,u_NPI,Wg_dot,D_dot,Lf] = fcn(S,e,xdot1,wr,Beta,wdotg,deltadot,Vdot,V,wg,delta,Pr,psihat,inte,DD,Wg,K,rd_hat)
ro=1.225;
R=35;
Jr=2.96e6;
Jg=53;
Ks=5.6e9;
Ds=1e7;
Ng=87.965;
taw=1;
Tg=8376.6;  
tau_beta=1;
landa=(wr*R)/(V);
landat=(1)/(landa+0.08*Beta)-0.035/(Beta^3+1);
% Cp=(0.22)*(116*landat-0.4*Beta-5)*(exp(-12.5*landat));
% Pr=0.5*pi*ro*R^2*V^3*Cp;

rf1_rx1=-(1/(Jr*wr))*(Pr/wr+0.11*pi*ro*R^3*V^2*((178.5-1450*landat+5*Beta)/((landa+0.08*Beta)^2))*(exp(-12.5*landat)))-Ds/Jr;
rf1_rx2=(Ds)/(Ng*Jr);
rf1_rx3=-Ks/Jr;
rf1_rx4=((0.11*pi*ro*R^2*V^3)/(wr*Jr))*((178.5-1450*landat+5*Beta)*((-0.08)/((landa+0.08*Beta)^2)+(0.105*Beta^2)/((Beta^3+1)^2))-0.4)*(exp(-12.5*landat));
rf1_rV=((0.11*pi*ro*R^3*V)/(Jr*(landa+0.08*Beta)^2))*(178.5-1450*landat+5*Beta)*(exp(-12.5*landat));

Lf=rf1_rx1*xdot1+rf1_rx2*wdotg+rf1_rx3*deltadot+rf1_rx4*(-Beta/taw)+rf1_rV*Vdot;
Lg=((0.11*pi*ro*R^2*V^3)/(wr*Jr*taw))*((178.5-1450*landat+5*Beta)*((-0.08)/((landa+0.08*Beta)^2)+(0.105*Beta^2)/((Beta^3+1)^2))-0.4)*(exp(-12.5*landat));

b0 = -0.04;Kp=6.3;Ki=0.26;
u_NPI = (1/b0)*(-(Kp+Ki*inte)*e-psihat);

% u_RL = -(1/(Lg))*YY;

landa=0.5;
S = -xdot1+landa*e + 0*rd_hat;   %(2.1428-wr) 
u_RL = -(1/(Lg))*(Lf+landa*xdot1+rd_hat+K*tanh(S));

Wg_dot = (wr*Ds)/(Ng*Jg)-(Wg*Ds)/(Ng^2*Jg)+(DD*Ks)/(Ng*Jg)-Tg/Jg;
D_dot = wr - Wg/Ng;

f = Lf + Lg*u_NPI;

== matlab function WT_FAST_09_07_2023_Afzalian/Pitch Controller/NN_SMC/s1 ==
  data: zhat1 input; zhat2 input; zhat3 input; z1 input; u input; zhatdot1 output; zhatdot2 output; zhatdot3 output
function [zhatdot1,zhatdot2,zhatdot3] = fcn(zhat1,zhat2,zhat3,z1,u)

sigma=0.5;
b0=-0.04;
h=0.001;
k01=1.2e+2;
k02=4.8e+3;
k03=80.4;

if abs(z1-zhat1)<=h
fal=(sigma^2/(h^(1-sigma)))*(z1-zhat1);
else
    fal=sign((z1-zhat1))*sigma^2*abs(z1-zhat1);
end

zhatdot1=zhat2+k01*(z1-zhat1);
zhatdot2=zhat3+b0*u+k02*fal;
zhatdot3=k03*(0.5^2/(h^(1-0.25)))*(z1-zhat1);

== matlab function WT_FAST_09_07_2023_Afzalian/Pitch Controller/NN_SMC/Observer1 ==
  data: a1 input; RMS_wr output
function RMS_wr  = fcn(a1)

RMS_wr = a1;

== matlab function WT_FAST_09_07_2023_Afzalian/Pitch Controller/NN_SMC/s4 ==
  data: t input; e1 input; ed input; W_ad output; W_cd output; W_a input; W_c input; alpha_hat output; S output; WW_a output; WW_c output; rho_U output; rho_L output; e output
function [W_ad,W_cd,alpha_hat,S,WW_a,WW_c,rho_U,rho_L,e]   = Weight(t,e1,ed,W_a,W_c)

% W = [w1;w2;w3;w4;w5];   w1,w2,w3,w4,w5
b=0.5;Gama=2.95;Lc= 0.05;L_a = 0.1;Ks=0.5; k1 = 1.5; 

% S = ed + Gama*e1;

%%%%%%%%%%%%%%%%%%%%%%%%%%%%%%%%%%%%%%%%%%%%%%%%%%%%%%%%%%%%%%%%%%%%%%%
%%
m = 1;
n= 1;
rho_0 = 1;
rho_inf = 0.1;
a = 0.05;
rho_U = (rho_0-rho_inf)*exp(-a*t)+rho_inf;
rho_dot_U = -a*(rho_0-rho_inf)*exp(-a*t);

b = 0.05;
rho_L = (rho_0-rho_inf)*exp(-b*t)+rho_inf;
rho_dot_L = -b*(rho_0-rho_inf)*exp(-b*t);

L = e1/rho_U;
VV = abs((m+L)./(n-L));
z = 0.5*(log(VV));

H = ((n*exp(z)-m*exp(-z))./(exp(z)+exp(-z)));

e = rho_U*H;

alpha = 0.5*(1/(e+rho_U)) + 0.5*(1/(rho_L-e));
beta = -0.5*(rho_dot_U/(e+rho_U))+0.5*(rho_dot_L/(e+rho_L));
zd = alpha*ed - beta;
landa = 5;
S = landa*z+2*zd';
%%%%%%%%%%%%%%%%%%%%%%%%%%%%%%%%%%%%%%%%%%%%%%%%%%%%%%%%%%%%%%%%%%%%%%%
%%
ZZ = norm(S);
zeta = exp(-(ZZ^2)/(2*b^2));
XX = -(ZZ/b^2)*zeta;
% k1 = -rho_U;

phi = -XX.*(Ks*e+0.5*XX.*W_a+0.5*(e/(k1^2-e^2)));
   
W_ad = (Ks*e+0.5*(e/(k1^2-e^2))).*XX-L_a*XX.*XX'.*W_a+(Lc/(1+(norm(phi))^2)).*XX.*XX'.*W_a.*phi.*W_c;

W_cd = -(Lc/(1+(norm(phi))^2)).*phi.*(phi'.*W_c-(Ks^2+Ks/(k1^2-e^2)).*(norm(e))^2 -(2*Ks.*e'+(e/(k1^2-e^2)).*0+0.25*(norm(XX'.*W_a))-(1/4)*(norm((e/(k1^2-e^2))))));
       
alpha_hat = -0.5*XX.*W_a-Ks*e-0.5*(e/(k1^2-e^2));

WW_c = norm(W_c);
WW_a = norm(W_a);

MM = (k1^2/(k1^2-e^2));

J1 = Ks*(norm(e))^2+W_c*zeta+0.5*log10(complex(MM));

end

== matlab function WT_FAST_09_07_2023_Afzalian/Pitch Controller/NN_SMC/D_hat ==
  data: dhat input; d input; bhat3 input; bhat3_dot output; dhat_dot output
function [bhat3_dot,dhat_dot] = Force(dhat,d,bhat3)


b1 = 10; b2 = 10; v = 0.1; h1 = 1.2; h2 = 0.8;

sa = d - dhat;
bhat3_dot = v*abs(sa);

dhat_dot = b1*(abs(sa)).^h1.*sign(sa)...
           +b2*(abs(sa)).^h2.*sign(sa)+bhat3.*sign(sa);

== matlab function WT_FAST_09_07_2023_Afzalian/Pitch Controller/NN_SMC/Observer2 ==
  data: u input; H output; t input; Wr input
function H  = fcn(u,t,Wr)

H = u + tanh(t-0.8) + Wr;

end

== matlab function WT_FAST_09_07_2023_Afzalian/Pitch Controller/NN_SMC/Observer4 ==
  data: a1 input; RMS_wr output
function RMS_wr  = fcn(a1)

RMS_wr = a1;

== matlab function WT_FAST_09_07_2023_Afzalian/s1 ==
  data: a1 input; a2 input; a3 input; a4 input; a5 input; RMS output; a6 input; a7 input; a8 input; a9 input
function RMS = fcn(a1,a2,a3,a4,a5,a6,a7,a8,a9)

RMS = [a1;a2;a3;a4;a5;a6;a7;a8;a9];

== matlab function WT_FAST_09_07_2023_Afzalian/Pitch Controller/NN_SMC/D_hat1 ==
  data: dhat input; d input; bhat3 input; bhat3_dot output; dhat_dot output
function [bhat3_dot,dhat_dot] = Force(dhat,d,bhat3)


b1 = 10; b2 = 10; v = 0.1; h1 = 1.2; h2 = 0.8;

sa = d - dhat;
bhat3_dot = v*abs(sa);

dhat_dot = b1*(abs(sa)).^h1.*sign(sa)...
           +b2*(abs(sa)).^h2.*sign(sa)+bhat3.*sign(sa);

== matlab function WT_FAST_09_07_2023_Afzalian/Pitch Controller/NN_SMC/s2 ==
  data: ed1 input; W_ad output; W_cd output; U_hat output; W_a input; W_c input; alpha_hat input; WW_a output; WW_c output; alpha_dot input; F_h input; J2 output
function [W_ad,W_cd,U_hat,WW_a,WW_c,J2]   = Weight(ed1,W_a,W_c,alpha_hat,alpha_dot,F_h)

% W = [w1;w2;w3;w4;w5];   w1,w2,w3,w4,w5
b=0.5;Lc= 0.05;L_a = 0.1;Ks2 = 0.008;k2 = 0.001;  

% S = ed + Gama*e;

e = ed1-alpha_hat;

ZZ = norm(e);
zeta = exp(-(ZZ^2)/(2*b^2));
XX = -(ZZ/b^2)*zeta;

phi = -XX.*(Ks2*e+0.5*XX.*W_a+0.5*(e/(k2^2-e^2))+(alpha_dot-F_h));
   
W_ad = (Ks2*e+0.5*(e/(k2^2-e^2))).*XX-L_a*XX.*XX'.*W_a+0.25*(Lc/(1+(norm(phi))^2)).*XX.*XX'.*W_a.*phi.*W_c;

W_cd = -(Lc/(1+(norm(phi))^2)).*phi.*(phi'.*W_c-(Ks2^2+Ks2/(k2^2-e^2)).*(norm(e))^2 -(2*Ks2.*e'+(e/(k2^2-e^2)).*(alpha_dot-F_h)+0.25*(norm(XX'.*W_a))-(1/4)*(norm((e/(k2^2-e^2))))));
       
U_hat = -0.5*XX.*W_a-Ks2*e-0.5*(e/(k2^2-e^2));

WW_c = norm(W_c);
WW_a = norm(W_a);

MM = (k2^2/(k2^2-e^2));
J2 = norm(Ks2*(norm(e))^2+W_c*zeta+0.5*log10(complex(MM)));



end

== matlab function WT_FAST_09_07_2023_Afzalian/Pitch Controller/NN_SMC/s3 ==
  data: eta input; eta_dot input; xdot1 input; e input; t input; Ka input; Ka_dot output; K output; Qh output; W output; Q output
function [Ka_dot,K,Qh,W,Q]  = Weight(eta,eta_dot,xdot1,e,t,Ka)

% W = [w1;w2;w3;w4;w5];   w1,w2,w3,w4,w5
landa = 0.5;
S = xdot1 + landa*e;

b=10.5;c=1;Gamma=10.5;a=0.05;ep=0.001;mu=0.6;yy=0.06;

ZZ = norm(e-c);
zeta = exp(-(ZZ^2)/(2*b^2));

zeta = zeta*ones(50,1);

% Rd = Gamma*(zeta*S-mu*W);

W = zeros(50,1);
dt = 0.0125;

for i = 1: 49
    W(i+1) = Gamma*(zeta(i)*S-mu*W(i))*dt + W(i);
end


Ka_dot = a*(abs(S)).^((5/3)-1)-yy*Ka;

% Ka_dot = a*(abs(S));

if t<=250
    K = Ka;
else
    K = abs(S)/(ep-abs(S));
end
Qh = W'*zeta;

landa=0.1;
Q = -eta_dot - landa*eta;
end
